simulink model "DP_SSR_LQR_PP"  (R2018b)
settings: Solver=ode45  StartTime=0.0  StopTime=6  RelTol=1e-3  EnableMultiTasking=on
InitFcn:
  | DP_code
values from neighbouring files (symbols this model uses):
  A = zeros(6,6)    [DP_code.m]    (also in IDP_code.m)
  B = zeros(6,1)    [DP_code.m]    (also in IDP_code.m)
  C = eye(6)    [DP_code.m]    (also in IDP_code.m)
  D = zeros(6,1)    [DP_code.m]    (also in IDP_code.m)
  K_lqr = lqr(A,B,Q,R)    [DP_code.m]    (also in IDP_code.m)
  K_pp_1 = place(A,B,P1)    [DP_code.m]    (also in IDP_code.m)
  K_pp_2 = place(A,B,P2)    [DP_code.m]    (also in IDP_code.m)
settings Model: Creator=user  LastModifiedBy=ahmed
settings DataIOCC: LimitDataPoints=on  SaveFormat=Array
settings OptimizationCC: LifeSpan=inf
settings DebuggingCC: UnderspecifiedInitializationDetection=Classic  MergeDetectMultiDrivingBlocksExec=none  SolverPrmCheckMsg=warning  StateNameClashWarn=warning  SFUnexpectedBacktrackingDiag=warning  SFNoUnconditionalDefaultTransitionDiag=warning  SFExecutionAtInitializationDiag=none
settings HardwareCC: ProdBitPerPointer=32  ProdBitPerSizeT=32  ProdBitPerPtrDiffT=32  ProdLargestAtomicFloat=None  ProdIntDivRoundTo=Undefined  ProdEndianess=Unspecified  ProdWordSize=32  ProdHWDeviceType=32-bit Generic
settings ModelReferenceCC: PropagateSignalLabelsOutOfModel=off
settings SFSimCC: SimUseLocalCustomCode=off
settings RTWCC: RTWUseLocalCustomCode=off
settings CodeAppCC: StateflowObjectComments=on
settings GRTTargetCC: TargetLangStandard=C89/C90 (ANSI)  GeneratePreprocessorConditionals=Disable all
settings ConfigComp: CovMetricSettings=dw  CovHtmlReporting=on  CovSaveCumulativeToWorkspaceVar=on  CovSaveSingleToWorkspaceVar=on  CovExternalEMLEnable=off

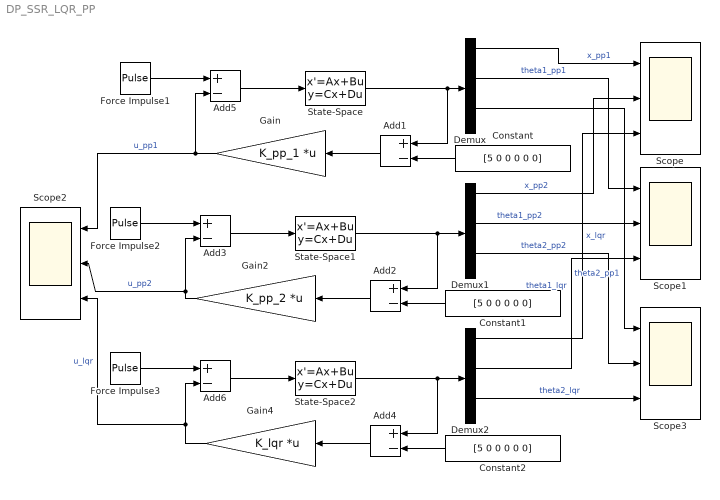
== system DP_SSR_LQR_PP ==
  Add{1..6} (6 alike) : Sum  Inputs=+-
  Constant : Constant  Value=[5 0 0 0 0 0]
  Constant1 : Constant  Value=[5 0 0 0 0 0]
  Constant2 : Constant  Value=[5 0 0 0 0 0]
  Demux : Demux  Outputs=6
  Demux1 : Demux  Outputs=6
  Demux2 : Demux  Outputs=6
  Force Impulse1 : DiscretePulseGenerator  PulseType=Time based  Amplitude=1000  Period=10  PulseWidth=0.01
  Force Impulse2 : DiscretePulseGenerator  PulseType=Time based  Amplitude=1000  Period=10  PulseWidth=0.01
  Force Impulse3 : DiscretePulseGenerator  PulseType=Time based  Amplitude=1000  Period=10  PulseWidth=0.01
  Gain : Gain  Gain=K_pp_1  Multiplication=Matrix(K*u) (u vector)
  Gain2 : Gain  Gain=K_pp_2  Multiplication=Matrix(K*u) (u vector)
  Gain4 : Gain  Gain=K_lqr  Multiplication=Matrix(K*u) (u vector)
  Scope{,1..3} (4 alike) : Scope  NumInputPorts=3
  State-Space : StateSpace  A=A  B=B  C=C  D=D  InitialCondition=0
  State-Space1 : StateSpace  A=A  B=B  C=C  D=D  InitialCondition=0
  State-Space2 : StateSpace  A=A  B=B  C=C  D=D  InitialCondition=0
  wires:
  Force Impulse1/1 -> Add5/1
  Add5/1 -> State-Space/1
  Gain/1 -> Scope2/1, Add5/2  "u_pp1"
  State-Space/1 -> Demux/1, Add1/1
  Add1/1 -> Gain/1
  Constant/1 -> Add1/2
  Force Impulse2/1 -> Add3/1
  Add3/1 -> State-Space1/1
  Gain2/1 -> Scope2/2, Add3/2  "u_pp2"
  State-Space1/1 -> Add2/1, Demux1/1
  Add2/1 -> Gain2/1
  Constant1/1 -> Add2/2
  Force Impulse3/1 -> Add6/1
  Add6/1 -> State-Space2/1
  Gain4/1 -> Scope2/3, Add6/2  "u_lqr"
  State-Space2/1 -> Add4/1, Demux2/1
  Add4/1 -> Gain4/1
  Constant2/1 -> Add4/2
  Demux/1 -> Scope/1  "x_pp1"
  Demux1/1 -> Scope/2  "x_pp2"
  Demux2/1 -> Scope/3  "x_lqr"
  Demux/3 -> Scope1/1  "theta1_pp1"
  Demux1/3 -> Scope1/2  "theta1_pp2"
  Demux2/3 -> Scope1/3  "theta1_lqr"
  Demux/5 -> Scope3/1  "theta2_pp1"
  Demux1/5 -> Scope3/2  "theta2_pp2"
  Demux2/5 -> Scope3/3  "theta2_lqr"
